simulink model "Copy_of_tests"  (R2024b)
settings: Solver=VariableStepAuto  StartTime=0.0  StopTime=1  RelTol=1e-3  AbsTol=1e-3  EnableMultiTasking=on
values from neighbouring files (symbols this model uses):
  m = obj.Br *obj.volume / obj.mu    [External_Magnet2.m]
  Params = Sim_Param_Setup    [Sim_Open.m]
undefined symbols (not defined in the file or in its folder): X, Y, Z
libraries: sm_lib x171, vrlib x144, nesl_utility x101, matrix_library x91, sharedtransform x12
(part 1 of 9)
settings Model: Creator=user  LastModifiedBy=user
settings SolverCC: AutoScaleAbsTol=off  AlgebraicLoopSolver=TrustRegion  MaxZcPerStep=1
settings DataIOCC: LimitDataPoints=on  MaxDataPoints=10000
settings OptimizationCC: ReuseModelBlockBuffer=off  LifeSpan=inf
settings DebuggingCC: UnconnectedInputMsg=warning  UnconnectedOutputMsg=warning  UnconnectedLineMsg=warning  AllowSymbolicDim=off  SubsystemReferenceDiagnosticForUnitTest=warning  SFUnexpectedBacktrackingDiag=warning  SFNoUnconditionalDefaultTransitionDiag=warning  SFExecutionAtInitializationDiag=none  ArithmeticOperatorsInVariantConditions=warning
settings ModelReferenceCC: EnableRefExpFcnMdlSchedulingChecks=on
settings SFSimCC: SimUseLocalCustomCode=off  CustomCodeUndefinedFunction=UseInterfaceOnly
settings RTWCC: RTWUseLocalCustomCode=off  GPUComputeCapability=3.5  DLArmComputeVersion=19.05
settings CodeAppCC: StateflowObjectComments=on
settings GRTTargetCC: TargetLangStandard=C89/C90 (ANSI)
settings ConfigComp: CovMetricSettings=dw  CovSaveCumulativeToWorkspaceVar=on  CovSaveSingleToWorkspaceVar=on  CovExternalEMLEnable=off  CovSFcnEnable=off
settings SimscapeCC: SimscapeLogType=all  SimscapeLogSimulationStatistics=on  SimscapeLogDataHistory=10000

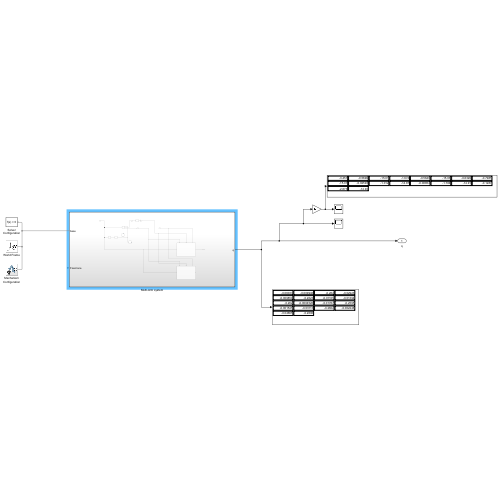
[thumbnail: Simulink's stored preview of the top-level diagram]
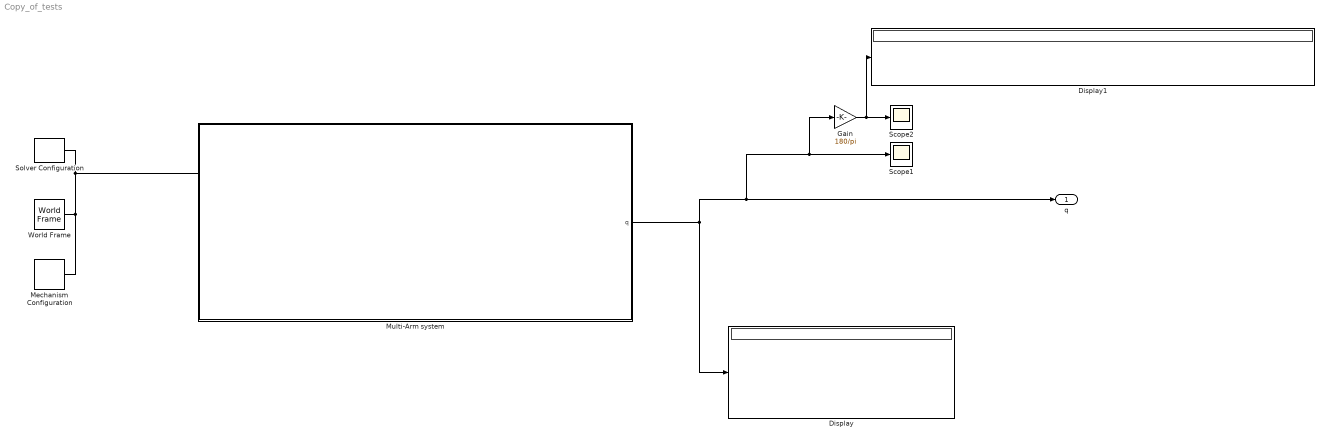
== system Copy_of_tests ==
  Display : Display
  Display1 : Display
  Gain : Gain  Gain=180/pi
  Mechanism Configuration : sm_lib/Utilities/Mechanism Configuration  UniformGravity=Constant  GravityVector=[0 -9.81 0]  GravityVectorUnits=m/s^2  LinearizationDelta=0.001  JointModeTransitionNonlinearIterations=2
  Multi-Arm system : Subsystem
  Scope1 : Scope
  Scope2 : Scope
  Solver Configuration : nesl_utility/Solver Configuration  PhysicalDomain=network_engine_domain  SubClassName=solver  LeftPortType=input  RightPortType=generic  Tones=[]  Harmonics=[]  SimulateNoise=off  Profile=off  UseLocalSampling=off  EnableSwitchedLinearOptims=on  FrequencyDomain=off  UseCCode=off  RelTol=0.001  AbsTol=1e-06  MinStep=1e-09  ToWorkspace=off  RevertToSquareIcSolve=off  NumHomotopyIterations=100  PhasorMode=off  PhasorModeNumHarmonics=1  ConsistencySolver=NEWTON_XTOL_AFTER_FTOL  IndexReductionMethod=DerivativeReplacement  DoDC=off  ResidualTolerance=1e-09  ConsistencyTolSource=GLOBAL  ConsistencyAbsTol=0.001  ConsistencyRelTol=0.001  ConsistencyTolFactor=0.001  UseLocalSolver=off  LocalSolverChoice=NE_BACKWARD_EULER_ADVANCER  ResolveIndetEquations=on  FunctionEvalNumThread=1  LocalSolverSampleTime=0.001  DoFixedCost=off  MaxNonlinIter=3  MaxModeIter=2  ComputeImpulses=off  ImpulseIterations=2  LinearAlgebra=Sparse  LinearAlgebraNumThread=0  EquationFormulation=NE_TIME_EF  DelaysMemoryBudget=1024  AutomaticFiltering=on  FilteringTimeConstant=0.001  PartitionStorageMethod=AS_NEEDED  PartitionMemoryBudget=1024  PartitionMethod=FAST  MultibodyUseLocalSolver=off  MultibodyLocalSolverChoice=ODE1  MultibodyLocalSolverSampleTime=0.001
  World Frame : sm_lib/Frames and Transforms/World Frame
  q : Outport
  wires:
  Gain/1 -> Display1/1, Scope2/1
  Multi-Arm system/1(q) -> Gain/1, Scope1/1, q/1, Display/1
  connections:
  Mechanism Configuration/RConn1 -- Solver Configuration/RConn1 -- Multi-Arm system/LConn1 -- World Frame/RConn1

== system Copy_of_tests/Multi-Arm system ==
  Brick Solid : sm_lib/Body Elements/Brick Solid  BrickDimensions=[5 20 20]  BrickDimensionsUnits=mm  ExportEntireGeometry=off  InertiaType=CalculateFromGeometry  BasedOnType=Density  Density=1000  DensityUnits=kg/m^3  Mass=1  MassUnits=kg  CenterOfMass=[0 0 0]  CenterOfMassUnits=m  MomentsOfInertia=[1 1 1]  MomentsOfInertiaUnits=kg*m^2  ProductsOfInertia=[0 0 0]  ProductsOfInertiaUnits=kg*m^2  GraphicType=FromGeometry  MarkerShape=Sphere  MarkerSize=10  GraphicVisPropType=SimpleVisualProperties  GraphicDiffuseColor=[1 0 0]  GraphicOpacity=1  GraphicSpecularColor=[0.5 0.5 0.5 1.0]  GraphicAmbientColor=[0.15 0.15 0.15 1.0]  GraphicEmissiveColor=[0.0 0.0 0.0 1.0]  GraphicShininess=75  DoExposeReferenceFrame=on  SerializedFrames=<Frames><Frame><Id>Frame1</Id><Value><Name>F1</Name><Origin><Source>GeometricFeature</Source><FeatureName>-x surface</FeatureName></Origin><PrimaryAxis><DefinedDirection>+Z</DefinedDirection><Source>ReferenceFrame</Source><SourceDirection>+Z</SourceDirection><FeatureName></FeatureName></PrimaryAxis><SecondaryAxis><DefinedDirection>+X</DefinedDirection><Source>ReferenceFrame</Source><SourceDirection>+X</SourceDirection><FeatureName></FeatureName></SecondaryAxis></Value></Frame><Frame><Id>Frame2</Id><Value><Name>F2</Name><Origin><Source>GeometricFeature</Source><FeatureName>+x surface</FeatureName></Origin><PrimaryAxis><DefinedDirection>+Z</DefinedDirection><Source>ReferenceFrame</Source><SourceDirection>+Z</SourceDirection><FeatureName></FeatureName></PrimaryAxis><SecondaryAxis><DefinedDirection>+X</DefinedDirection><Source>ReferenceFrame</Source><SourceDirection>+X</SourceDirection><FeatureName></FeatureName></SecondaryAxis></Value></Frame></Frames>
  Brick Solid1 : sm_lib/Body Elements/Brick Solid  BrickDimensions=[5 20 20]  BrickDimensionsUnits=mm  ExportEntireGeometry=off  InertiaType=CalculateFromGeometry  BasedOnType=Density  Density=1000  DensityUnits=kg/m^3  Mass=1  MassUnits=kg  CenterOfMass=[0 0 0]  CenterOfMassUnits=m  MomentsOfInertia=[1 1 1]  MomentsOfInertiaUnits=kg*m^2  ProductsOfInertia=[0 0 0]  ProductsOfInertiaUnits=kg*m^2  GraphicType=FromGeometry  MarkerShape=Sphere  MarkerSize=10  GraphicVisPropType=SimpleVisualProperties  GraphicDiffuseColor=[0 0 1]  GraphicOpacity=1  GraphicSpecularColor=[0.5 0.5 0.5 1.0]  GraphicAmbientColor=[0.15 0.15 0.15 1.0]  GraphicEmissiveColor=[0.0 0.0 0.0 1.0]  GraphicShininess=75  DoExposeReferenceFrame=on  SerializedFrames=<Frames><Frame><Id>Frame1</Id><Value><Name>F1</Name><Origin><Source>GeometricFeature</Source><FeatureName>-x surface</FeatureName></Origin><PrimaryAxis><DefinedDirection>+Z</DefinedDirection><Source>ReferenceFrame</Source><SourceDirection>+Z</SourceDirection><FeatureName></FeatureName></PrimaryAxis><SecondaryAxis><DefinedDirection>+X</DefinedDirection><Source>ReferenceFrame</Source><SourceDirection>+X</SourceDirection><FeatureName></FeatureName></SecondaryAxis></Value></Frame></Frames>
  Gain1 : Gain  Gain=-1*Params.Source_MagnetMagnitude
  PS-Simulink Converter : nesl_utility/PS-Simulink Converter  PhysicalDomain=network_engine_domain  SubClassName=ps_output  LeftPortType=input  RightPortType=output  PseudoPeriodic=off  Frequencies=[]  VectorFormat=inherit  Unit=inherit  AffineConversion=off
  PS-Simulink Converter1 : nesl_utility/PS-Simulink Converter  PhysicalDomain=network_engine_domain  SubClassName=ps_output  LeftPortType=input  RightPortType=output  PseudoPeriodic=off  Frequencies=[]  VectorFormat=inherit  Unit=inherit  AffineConversion=off
  Rigid Transform1 : sm_lib/Frames and Transforms/Rigid Transform  RotationMethod=None  FollAlignAxisA=+X  BaseAlignAxisA=+Y  FollAlignAxisB=+Y  BaseAlignAxisB=+Z  RotationStandardAxis=+Z  RotationAngle=0.0  RotationAngleUnits=deg  RotationArbitraryAxis=[0 0 1]  RotationSequenceAxes=FollowerAxes  RotationSequence=XYX  RotationSequenceAngles=[0 0 0]  RotationSequenceAnglesUnits=deg  RotationMatrix=[1 0 0; 0 1 0; 0 0 1]  Quaternion=[1 0 0 0]  TranslationMethod=Cartesian  TranslationCartesianOffset=[Params.Source_Distance_x Params.Source_Distance_y 0]  TranslationCartesianOffsetUnits=m  TranslationStandardAxis=+X  TranslationStandardOffset=0.1e-3  TranslationStandardOffsetUnits=m  TranslationROffset=0  TranslationROffsetUnits=m  TranslationThetaOffset=0  TranslationThetaOffsetUnits=deg  TranslationZOffset=0  TranslationZOffsetUnits=m
  Rigid Transform2 : sm_lib/Frames and Transforms/Rigid Transform  RotationMethod=StandardAxis  FollAlignAxisA=+X  BaseAlignAxisA=+Y  FollAlignAxisB=+Y  BaseAlignAxisB=+Z  RotationStandardAxis=+Z  RotationAngle=Params.Source_Angle  RotationAngleUnits=deg  RotationArbitraryAxis=[0 0 1]  RotationSequenceAxes=FollowerAxes  RotationSequence=XYX  RotationSequenceAngles=[0 0 0]  RotationSequenceAnglesUnits=deg  RotationMatrix=[1 0 0; 0 1 0; 0 0 1]  Quaternion=[1 0 0 0]  TranslationMethod=None  TranslationCartesianOffset=[Params.Source_Distance_x Params.Source_Distance_y 0]  TranslationCartesianOffsetUnits=m  TranslationStandardAxis=+X  TranslationStandardOffset=0.1e-3  TranslationStandardOffsetUnits=m  TranslationROffset=0  TranslationROffsetUnits=m  TranslationThetaOffset=0  TranslationThetaOffsetUnits=deg  TranslationZOffset=0  TranslationZOffsetUnits=m
  Single_Arm 1 : Subsystem
      settings: PortSchema="{\"entries\":[{\"content\":{\"sides\":[{\"content\":{\"connectorIds\":[\"Out1\"]},\"type\":\"ConnectorPlacement.EquallySpacedRectSide\",\"uuid\":\"aed73cf6-d05b-4742-919d-2a5b7405f7c0\"},{\"content\":{\"connectorIds\":[\"RConn1\"],\"side\":\"RIGHT\"},\"type\":\"ConnectorPlacement.EquallySpacedRectSide\",\"uuid\":\"b6800f08-4bd8-49f5-86ab-f689441aa6b5\"},{\"content\":{\"connectorIds\":[\"LConn1\",\"In1\",\"In2\"],\"side\":\"TOP\"},\"type\":\"ConnectorPlacement.EquallySpacedRectSide\",\"uuid\":\"ec4c69cc-0faf-459d-a169-37761ab2dd6d\"},{\"content\":{\"side\":\"BOTTOM\"},\"type\":\"ConnectorPlacement.EquallySpacedRectSide\",\"uuid\":\"2a21d102-aa49-4e33-81c3-df43061c4ef1\"}]},\"type\":\"ConnectorPlacement.EquallySpacedConnector\",\"uuid\":\"838f12d2-4917-4325-9f22-e0bcefcce707\"}],\"packageUris\":[\"http://schema.mathworks.com/mf0/Connector/R2020b\"],\"version\":\"1.0\"}"
  Single_Arm 2 : Subsystem
      settings: PortSchema="{\"entries\":[{\"content\":{\"sides\":[{\"content\":{\"connectorIds\":[\"Out1\"]},\"type\":\"ConnectorPlacement.EquallySpacedRectSide\",\"uuid\":\"aed73cf6-d05b-4742-919d-2a5b7405f7c0\"},{\"content\":{\"connectorIds\":[\"RConn1\"],\"side\":\"RIGHT\"},\"type\":\"ConnectorPlacement.EquallySpacedRectSide\",\"uuid\":\"b6800f08-4bd8-49f5-86ab-f689441aa6b5\"},{\"content\":{\"connectorIds\":[\"LConn1\",\"In1\",\"In2\"],\"side\":\"TOP\"},\"type\":\"ConnectorPlacement.EquallySpacedRectSide\",\"uuid\":\"ec4c69cc-0faf-459d-a169-37761ab2dd6d\"},{\"content\":{\"side\":\"BOTTOM\"},\"type\":\"ConnectorPlacement.EquallySpacedRectSide\",\"uuid\":\"2a21d102-aa49-4e33-81c3-df43061c4ef1\"}]},\"type\":\"ConnectorPlacement.EquallySpacedConnector\",\"uuid\":\"838f12d2-4917-4325-9f22-e0bcefcce707\"}],\"packageUris\":[\"http://schema.mathworks.com/mf0/Connector/R2020b\"],\"version\":\"1.0\"}"
  Submatrix : matrix_library/Submatrix  RowSpan=Range of rows  RowStartMode=First  RowStartIndex=1  RowEndMode=Last  RowEndIndex=1  ColSpan=One column  ColStartMode=First  ColStartIndex=1  ColEndMode=Last  ColEndIndex=1
  Transform Sensor : sm_lib/Frames and Transforms/Transform Sensor  MeasurementFrame=Base  RotationSequence=XYX  SenseAngle=off  SenseAxis=off  SenseQ=off  SenseR=on  SenseRotationSequence=off  SenseOmegaX=off  SenseOmegaY=off  SenseOmegaZ=off  SenseOmega=off  SenseQDot=off  SenseRDot=off  SenseRotationSequenceDot=off  SenseAlphaX=off  SenseAlphaY=off  SenseAlphaZ=off  SenseAlpha=off  SenseQDDot=off  SenseRDDot=off  SenseX=off  SenseY=off  SenseZ=off  SenseXYZ=on  SenseRad=off  SenseAzim=off  SenseDist=off  SenseInc=off  SenseXDot=off  SenseYDot=off  SenseZDot=off  SenseXYZDot=off  SenseRadDot=off  SenseAzimDot=off  SenseDistDot=off  SenseIncDot=off  SenseXDDot=off  SenseYDDot=off  SenseZDDot=off  SenseXYZDDot=off  SenseRadDDot=off  SenseAzimDDot=off  SenseDistDDot=off  SenseIncDDot=off
  base : PMIOPort  Side=Left
  Fixed one : PMIOPort  Port=2  Side=Left
  q : Outport
  wires:
  PS-Simulink Converter1/1 -> Submatrix/1
  Gain1/1 -> Single_Arm 1/1(Source_Moment), Single_Arm 2/1(Source_Moment)
  Submatrix/1 -> Gain1/1
  Single_Arm 1/1(q) -> q/1
  PS-Simulink Converter/1 -> Single_Arm 1/2(Source_Pos), Single_Arm 2/2(Source_Pos)
  connections:
  Brick Solid/LConn2 -- Transform Sensor/RConn1 -- Brick Solid1/LConn1
  Rigid Transform1/RConn1 -- Rigid Transform2/LConn1
  Rigid Transform2/RConn1 -- Brick Solid/LConn1
  Single_Arm 1/LConn1 -- Fixed one/RConn1 -- Single_Arm 2/LConn1
  base/RConn1 -- Single_Arm 2/RConn1 -- Single_Arm 1/RConn1 -- Rigid Transform1/LConn1 -- Transform Sensor/LConn1
  Transform Sensor/RConn3 -- PS-Simulink Converter/LConn1
  PS-Simulink Converter1/LConn1 -- Transform Sensor/RConn2

== system Copy_of_tests/Multi-Arm system/Single_Arm 1 ==
  Source_Moment : Inport
  Source_Pos : Inport  Port=2
  Mux : Mux  Inputs=6
  PS-Simulink Converter{,1..5} (6 alike) : nesl_utility/PS-Simulink Converter  PhysicalDomain=network_engine_domain  SubClassName=ps_output  LeftPortType=input  RightPortType=output  PseudoPeriodic=off  Frequencies=[]  VectorFormat=inherit  Unit=inherit  AffineConversion=off
  Plate_0 : Subsystem
  Plate_1 : Subsystem
      settings: PortSchema="{\"entries\":[{\"content\":{\"sides\":[{\"content\":{\"connectorIds\":[\"LConn1\"]},\"type\":\"ConnectorPlacement.EquallySpacedRectSide\",\"uuid\":\"d3209e73-b1b0-400d-bb69-5c2c223e1cf5\"},{\"content\":{\"connectorIds\":[\"RConn1\"],\"side\":\"RIGHT\"},\"type\":\"ConnectorPlacement.EquallySpacedRectSide\",\"uuid\":\"f1a30951-4015-44b6-8cd5-c465137d5200\"},{\"content\":{\"connectorIds\":[\"In1\",\"In2\",\"In3\",\"In4\",\"In5\",\"In6\",\"In7\",\"In8\",\"In9\",\"In10\",\"Out1\",\"Out2\"],\"side\":\"TOP\"},\"type\":\"ConnectorPlacement.EquallySpacedRectSide\",\"uuid\":\"858e4eb2-ea22-4c31-a0a7-90acc6749235\"},{\"content\":{\"connectorIds\":[\"In11\",\"In12\"],\"side\":\"BOTTOM\"},\"type\":\"ConnectorPlacement.EquallySpacedRectSide\",\"uuid\":\"4614ed4f-637f-4a9b-aac4-e5064df79866\"}]},\"type\":\"ConnectorPlacement.EquallySpacedConnector\",\"uuid\":\"0376ba42-8dd9-4ddf-9e80-cb6449970d36\"}],\"packageUris\":[\"http://schema.mathworks.com/mf0/Connector/R2020b\"],\"version\":\"1.0\"}"
  Plate_2 : Subsystem
      settings: PortSchema="{\"entries\":[{\"content\":{\"sides\":[{\"content\":{\"connectorIds\":[\"LConn1\"]},\"type\":\"ConnectorPlacement.EquallySpacedRectSide\",\"uuid\":\"ec18759c-59e4-4a78-8a02-c5f79d16e625\"},{\"content\":{\"connectorIds\":[\"RConn1\"],\"side\":\"RIGHT\"},\"type\":\"ConnectorPlacement.EquallySpacedRectSide\",\"uuid\":\"7dbb223b-0b69-4dcf-bc3d-f54c7924a0b4\"},{\"content\":{\"connectorIds\":[\"In1\",\"In2\",\"In3\",\"In4\",\"In5\",\"In6\",\"In7\",\"In8\",\"Out1\",\"Out2\",\"In9\",\"In10\"],\"side\":\"TOP\"},\"type\":\"ConnectorPlacement.EquallySpacedRectSide\",\"uuid\":\"897f1654-1cd8-4ed9-9f75-2958da94a55c\"},{\"content\":{\"connectorIds\":[\"In11\",\"In12\"],\"side\":\"BOTTOM\"},\"type\":\"ConnectorPlacement.EquallySpacedRectSide\",\"uuid\":\"7ed320ae-75a8-4e52-84a2-f6626d5c5d01\"}]},\"type\":\"ConnectorPlacement.EquallySpacedConnector\",\"uuid\":\"b5c764c2-43a6-4160-9b0c-e997344b52fc\"}],\"packageUris\":[\"http://schema.mathworks.com/mf0/Connector/R2020b\"],\"version\":\"1.0\"}"
  Plate_3 : Subsystem
      settings: PortSchema="{\"entries\":[{\"content\":{\"sides\":[{\"content\":{\"connectorIds\":[\"LConn1\"]},\"type\":\"ConnectorPlacement.EquallySpacedRectSide\",\"uuid\":\"659d4c74-debd-4236-880d-faa78149b6ae\"},{\"content\":{\"connectorIds\":[\"RConn1\"],\"side\":\"RIGHT\"},\"type\":\"ConnectorPlacement.EquallySpacedRectSide\",\"uuid\":\"7acc4d0a-33e4-40af-a3d8-89f29cefab0d\"},{\"content\":{\"connectorIds\":[\"In1\",\"In2\",\"In3\",\"In4\",\"In5\",\"In6\",\"Out1\",\"Out2\",\"In7\",\"In8\",\"In9\",\"In10\"],\"side\":\"TOP\"},\"type\":\"ConnectorPlacement.EquallySpacedRectSide\",\"uuid\":\"3f8fe647-c128-4da8-9892-2ef747b61f38\"},{\"content\":{\"connectorIds\":[\"In11\",\"In12\"],\"side\":\"BOTTOM\"},\"type\":\"ConnectorPlacement.EquallySpacedRectSide\",\"uuid\":\"9ec47aaa-5f22-4f0a-90c6-c481dcf8db46\"}]},\"type\":\"ConnectorPlacement.EquallySpacedConnector\",\"uuid\":\"1b26417e-b7bd-4e51-87e9-74b02b81f54b\"}],\"packageUris\":[\"http://schema.mathworks.com/mf0/Connector/R2020b\"],\"version\":\"1.0\"}"
  Plate_4 : Subsystem
      settings: PortSchema="{\"entries\":[{\"content\":{\"sides\":[{\"content\":{\"connectorIds\":[\"LConn1\"]},\"type\":\"ConnectorPlacement.EquallySpacedRectSide\",\"uuid\":\"ec18759c-59e4-4a78-8a02-c5f79d16e625\"},{\"content\":{\"connectorIds\":[\"RConn1\"],\"side\":\"RIGHT\"},\"type\":\"ConnectorPlacement.EquallySpacedRectSide\",\"uuid\":\"7dbb223b-0b69-4dcf-bc3d-f54c7924a0b4\"},{\"content\":{\"connectorIds\":[\"In1\",\"In2\",\"In3\",\"In4\",\"Out1\",\"Out2\",\"In5\",\"In6\",\"In7\",\"In8\",\"In9\",\"In10\"],\"side\":\"TOP\"},\"type\":\"ConnectorPlacement.EquallySpacedRectSide\",\"uuid\":\"897f1654-1cd8-4ed9-9f75-2958da94a55c\"},{\"content\":{\"connectorIds\":[\"In11\",\"In12\"],\"side\":\"BOTTOM\"},\"type\":\"ConnectorPlacement.EquallySpacedRectSide\",\"uuid\":\"3c262aa2-4d18-4ec5-8376-adcb010a8e7d\"}]},\"type\":\"ConnectorPlacement.EquallySpacedConnector\",\"uuid\":\"b5c764c2-43a6-4160-9b0c-e997344b52fc\"}],\"packageUris\":[\"http://schema.mathworks.com/mf0/Connector/R2020b\"],\"version\":\"1.0\"}"
  Plate_5 : Subsystem
      settings: PortSchema="{\"entries\":[{\"content\":{\"sides\":[{\"content\":{\"connectorIds\":[\"LConn1\"]},\"type\":\"ConnectorPlacement.EquallySpacedRectSide\",\"uuid\":\"ec18759c-59e4-4a78-8a02-c5f79d16e625\"},{\"content\":{\"connectorIds\":[\"RConn1\"],\"side\":\"RIGHT\"},\"type\":\"ConnectorPlacement.EquallySpacedRectSide\",\"uuid\":\"7dbb223b-0b69-4dcf-bc3d-f54c7924a0b4\"},{\"content\":{\"connectorIds\":[\"In1\",\"In2\",\"Out1\",\"Out2\",\"In3\",\"In4\",\"In5\",\"In6\",\"In7\",\"In8\",\"In9\",\"In10\"],\"side\":\"TOP\"},\"type\":\"ConnectorPlacement.EquallySpacedRectSide\",\"uuid\":\"897f1654-1cd8-4ed9-9f75-2958da94a55c\"},{\"content\":{\"connectorIds\":[\"In11\",\"In12\"],\"side\":\"BOTTOM\"},\"type\":\"ConnectorPlacement.EquallySpacedRectSide\",\"uuid\":\"5987a4f9-0df9-407c-b6e6-a076c5272fc6\"}]},\"type\":\"ConnectorPlacement.EquallySpacedConnector\",\"uuid\":\"b5c764c2-43a6-4160-9b0c-e997344b52fc\"}],\"packageUris\":[\"http://schema.mathworks.com/mf0/Connector/R2020b\"],\"version\":\"1.0\"}"
  Plate_6 : Subsystem
      settings: PortSchema="{\"entries\":[{\"content\":{\"sides\":[{\"content\":{\"connectorIds\":[\"LConn1\"]},\"type\":\"ConnectorPlacement.EquallySpacedRectSide\",\"uuid\":\"ec18759c-59e4-4a78-8a02-c5f79d16e625\"},{\"content\":{\"connectorIds\":[\"RConn1\"],\"side\":\"RIGHT\"},\"type\":\"ConnectorPlacement.EquallySpacedRectSide\",\"uuid\":\"7dbb223b-0b69-4dcf-bc3d-f54c7924a0b4\"},{\"content\":{\"connectorIds\":[\"Out1\",\"Out2\",\"In1\",\"In2\",\"In3\",\"In4\",\"In5\",\"In6\",\"In7\",\"In8\",\"In9\",\"In10\"],\"side\":\"TOP\"},\"type\":\"ConnectorPlacement.EquallySpacedRectSide\",\"uuid\":\"897f1654-1cd8-4ed9-9f75-2958da94a55c\"},{\"content\":{\"connectorIds\":[\"In11\",\"In12\"],\"side\":\"BOTTOM\"},\"type\":\"ConnectorPlacement.EquallySpacedRectSide\",\"uuid\":\"c3ba0d0a-cbda-4d2d-b1e9-4fbf79d48483\"}]},\"type\":\"ConnectorPlacement.EquallySpacedConnector\",\"uuid\":\"b5c764c2-43a6-4160-9b0c-e997344b52fc\"}],\"packageUris\":[\"http://schema.mathworks.com/mf0/Connector/R2020b\"],\"version\":\"1.0\"}"
  Quaternions to Rotation Angles{,1..5} (6 alike) : sharedtransform/Quaternions to Rotation Angles  rotationOrder=ZYX  aMode=aMode
  Rigid Transform{1..12} (12 alike) : sm_lib/Frames and Transforms/Rigid Transform  RotationMethod=None  FollAlignAxisA=+X  BaseAlignAxisA=+Y  FollAlignAxisB=+Y  BaseAlignAxisB=+Z  RotationStandardAxis=+Z  RotationAngle=0.0  RotationAngleUnits=deg  RotationArbitraryAxis=[0 0 1]  RotationSequenceAxes=FollowerAxes  RotationSequence=XYX  RotationSequenceAngles=[0 0 0]  RotationSequenceAnglesUnits=deg  RotationMatrix=[1 0 0; 0 1 0; 0 0 1]  Quaternion=[1 0 0 0]  TranslationMethod=StandardAxis  TranslationCartesianOffset=[0 0 0]  TranslationCartesianOffsetUnits=m  TranslationStandardAxis=+X  TranslationStandardOffset=0.1e-3  TranslationStandardOffsetUnits=m  TranslationROffset=0  TranslationROffsetUnits=m  TranslationThetaOffset=0  TranslationThetaOffsetUnits=deg  TranslationZOffset=0  TranslationZOffsetUnits=m
  Spherical Joint{,1..5} (6 alike) : sm_lib/Joints/Spherical Joint  JointMode=Normal  CompositeWrenchDir=FollowerOnBase  CompositeWrenchFrame=BaseFrame  SenseConstraintForce=off  SenseConstraintTorque=off  SenseTotalForce=off  SenseTotalTorque=off  PositionTargetSpecify=off  PositionTargetPriority=High  PositionTargetRotationMethod=None  PositionTargetFollAlignAxisA=+X  PositionTargetBaseAlignAxisA=+Y  PositionTargetFollAlignAxisB=+Y  PositionTargetBaseAlignAxisB=+Z  PositionTargetRotationStandardAxis=+Z  PositionTargetRotationAngle=0  PositionTargetRotationAngleUnits=deg  PositionTargetRotationArbitraryAxis=[0 0 1]  PositionTargetRotationSequenceAxes=FollowerAxes  PositionTargetRotationSequence=XYX  PositionTargetRotationSequenceAngles=[0 0 0]  PositionTargetRotationSequenceAnglesUnits=deg  PositionTargetRotationMatrix=[1 0 0;0 1 0;0 0 1]  PositionTargetQuaternion=[1 0 0 0]  VelocityTargetSpecify=off  VelocityTargetPriority=High  VelocityTargetValue=[0 0 0]  VelocityTargetValueUnits=deg/s  VelocityTargetInFollowerFrame=on  EqPosRotationMethod=None  EqPosFollAlignAxisA=+X  EqPosBaseAlignAxisA=+Y  EqPosFollAlignAxisB=+Y  EqPosBaseAlignAxisB=+Z  EqPosRotationStandardAxis=+Z  EqPosRotationAngle=0  EqPosRotationAngleUnits=deg  EqPosRotationArbitraryAxis=[0 0 1]  EqPosRotationSequenceAxes=FollowerAxes  EqPosRotationSequence=XYX  EqPosRotationSequenceAngles=[0 0 0]  EqPosRotationSequenceAnglesUnits=deg  EqPosRotationMatrix=[1 0 0;0 1 0;0 0 1]  EqPosQuaternion=[1 0 0 0]  SpringStiffness=Params.Stiffness  SpringStiffnessUnits=N*m/deg  DampingCoefficient=Params.Damping  DampingCoefficientUnits=N*m/(deg/s)  LowerLimitSpecify=off  LowerLimitBound=15  LowerLimitBoundUnits=deg  LowerLimitStiffness=1e4  LowerLimitStiffnessUnits=N*m/deg  LowerLimitDamping=10  LowerLimitDampingUnits=N*m/(deg/s)  LowerLimitTransitionRegionWidth=0.1  LowerLimitTransitionRegionWidthUnits=deg  UpperLimitSpecify=off  UpperLimitBound=45  UpperLimitBoundUnits=deg  UpperLimitStiffness=1e4  UpperLimitStiffnessUnits=N*m/deg  UpperLimitDamping=10  UpperLimitDampingUnits=N*m/(deg/s)  UpperLimitTransitionRegionWidth=0.1  UpperLimitTransitionRegionWidthUnits=deg  TorqueActuationMode=NoTorque  ActuateTorqueX=off  ActuateTorqueY=off  ActuateTorqueZ=off  ActuateTorque=off  ActuationFrame=BaseFrame  SensePosition=on  SenseVelocityX=off  SenseVelocityY=off  SenseVelocityZ=off  SenseVelocity=off  SenseAccelerationX=off  SenseAccelerationY=off  SenseAccelerationZ=off  SenseAcceleration=off  SenseLowerLimitTorqueMag=off  SenseUpperLimitTorqueMag=off  SensingFrame=BaseFrame
  Fixed one : PMIOPort  Side=Left
  base : PMIOPort  Port=2  Side=Right
  q : Outport
  wires:
  PS-Simulink Converter/1 -> Quaternions to Rotation Angles/1
  PS-Simulink Converter1/1 -> Quaternions to Rotation Angles1/1
  PS-Simulink Converter2/1 -> Quaternions to Rotation Angles2/1
  PS-Simulink Converter3/1 -> Quaternions to Rotation Angles3/1
  PS-Simulink Converter5/1 -> Quaternions to Rotation Angles5/1
  PS-Simulink Converter4/1 -> Quaternions to Rotation Angles4/1
  Mux/1 -> q/1
  Plate_2/1(Pos_Plate2) -> Plate_6/7(Pos_Plate2), Plate_5/7(Pos_Plate2), Plate_4/7(Pos_Plate2), Plate_3/7(Pos_Plate2), Plate_1/9(Pos_Plate2)
  Plate_2/2(M2) -> Plate_6/8(M2), Plate_5/8(M2), Plate_4/8(M2), Plate_3/8(M2), Plate_1/10(M2)
  Plate_1/2(M1) -> Plate_6/10(M1), Plate_5/10(M1), Plate_4/10(M1), Plate_3/10(M1), Plate_2/10(M1)
  Plate_1/1(Pos_Plate1) -> Plate_6/9(Pos_Plate1), Plate_5/9(Pos_Plate1), Plate_4/9(Pos_Plate1), Plate_3/9(Pos_Plate1), Plate_2/9(Pos_Plate1)
  Plate_3/2(M3) -> Plate_6/6(M3), Plate_5/6(M3), Plate_4/6(M3), Plate_2/8(M3), Plate_1/8(M3)
  Plate_3/1(Pos_Plate3) -> Plate_6/5(Pos_Plate3), Plate_5/5(Pos_Plate3), Plate_4/5(Pos_Plate3), Plate_2/7(Pos_Plate3), Plate_1/7(Pos_Plate3)
  Plate_4/2(M4) -> Plate_6/4(M4), Plate_5/4(M4), Plate_3/6(M4), Plate_2/6(M4), Plate_1/6(M4)
  Plate_4/1(Pos_Plate4) -> Plate_6/3(Pos_Plate4), Plate_5/3(Pos_Plate4), Plate_3/5(Pos_Plate4), Plate_2/5(Pos_Plate4), Plate_1/5(Pos_Plate4)
  Plate_5/2(M5) -> Plate_6/2(M5), Plate_4/4(M5), Plate_3/4(M5), Plate_2/4(M5), Plate_1/4(M5)
  Plate_5/1(Pos_Plate5) -> Plate_6/1(Pos_Plate5), Plate_4/3(Pos_Plate5), Plate_3/3(Pos_Plate5), Plate_2/3(Pos_Plate5), Plate_1/3(Pos_Plate5)
  Plate_6/2(M6) -> Plate_5/2(M6), Plate_4/2(M6), Plate_3/2(M6), Plate_2/2(M6), Plate_1/2(M6)
  Plate_6/1(Pos_Plate6) -> Plate_5/1(Pos_Plate6), Plate_4/1(Pos_Plate6), Plate_3/1(Pos_Plate6), Plate_2/1(Pos_Plate6), Plate_1/1(Pos_Plate6)
  Quaternions to Rotation Angles/1 -> Mux/1
  Quaternions to Rotation Angles1/1 -> Mux/2
  Quaternions to Rotation Angles2/1 -> Mux/3
  Quaternions to Rotation Angles3/1 -> Mux/4
  Quaternions to Rotation Angles4/1 -> Mux/5
  Quaternions to Rotation Angles5/1 -> Mux/6
  Source_Moment/1 -> Plate_6/12(Source_Moment), Plate_5/12(Source_Moment), Plate_4/12(Source_Moment), Plate_3/12(Source_Moment), Plate_2/12(Source_Moment), Plate_1/12(Source_Moment)
  Source_Pos/1 -> Plate_6/11(Source_Pos), Plate_5/11(Source_Pos), Plate_4/11(Source_Pos), Plate_3/11(Source_Pos), Plate_2/11(Source_Pos), Plate_1/11(Source_Pos)
  connections:
  Rigid Transform11/RConn1 -- Plate_6/RConn1
  Spherical Joint1/LConn1 -- Rigid Transform3/RConn1
  Spherical Joint5/LConn1 -- Rigid Transform12/RConn1
  Rigid Transform2/LConn1 -- Spherical Joint/RConn1
  Rigid Transform11/LConn1 -- Spherical Joint5/RConn1
  Rigid Transform10/RConn1 -- Plate_5/RConn1
  Rigid Transform10/LConn1 -- Spherical Joint4/RConn1
  Rigid Transform4/LConn1 -- Spherical Joint1/RConn1
  Rigid Transform8/RConn1 -- Plate_4/RConn1
  Spherical Joint4/LConn1 -- Rigid Transform9/RConn1
  Plate_4/LConn1 -- Rigid Transform9/LConn1
  Spherical Joint3/LConn1 -- Rigid Transform7/RConn1
  Rigid Transform6/RConn1 -- Plate_3/RConn1
  Rigid Transform8/LConn1 -- Spherical Joint3/RConn1
  Plate_3/LConn1 -- Rigid Transform7/LConn1
  Plate_0/LConn1 -- Rigid Transform1/LConn1
  Spherical Joint/LConn1 -- Rigid Transform1/RConn1
  Plate_2/LConn1 -- Rigid Transform5/LConn1
  Plate_1/LConn1 -- Rigid Transform3/LConn1
  Plate_5/LConn1 -- Rigid Transform12/LConn1
  Rigid Transform4/RConn1 -- Plate_2/RConn1
  Spherical Joint2/LConn1 -- Rigid Transform5/RConn1
  Rigid Transform6/LConn1 -- Spherical Joint2/RConn1
  Rigid Transform2/RConn1 -- Plate_1/RConn1
  Plate_6/LConn1 -- Fixed one/RConn1
  base/RConn1 -- Plate_0/RConn1
  Spherical Joint/RConn2 -- PS-Simulink Converter/LConn1
  Spherical Joint1/RConn2 -- PS-Simulink Converter1/LConn1
  Spherical Joint2/RConn2 -- PS-Simulink Converter2/LConn1
  Spherical Joint3/RConn2 -- PS-Simulink Converter3/LConn1
  Spherical Joint4/RConn2 -- PS-Simulink Converter4/LConn1
  Spherical Joint5/RConn2 -- PS-Simulink Converter5/LConn1

== system Copy_of_tests/Multi-Arm system/Single_Arm 2 ==
  Source_Moment : Inport
  Source_Pos : Inport  Port=2
  Mux : Mux  Inputs=6
  PS-Simulink Converter{,1..5} (6 alike) : nesl_utility/PS-Simulink Converter  PhysicalDomain=network_engine_domain  SubClassName=ps_output  LeftPortType=input  RightPortType=output  PseudoPeriodic=off  Frequencies=[]  VectorFormat=inherit  Unit=inherit  AffineConversion=off
  Plate_0 : Subsystem
  Plate_1 : Subsystem
      settings: PortSchema="{\"entries\":[{\"content\":{\"sides\":[{\"content\":{\"connectorIds\":[\"LConn1\"]},\"type\":\"ConnectorPlacement.EquallySpacedRectSide\",\"uuid\":\"d3209e73-b1b0-400d-bb69-5c2c223e1cf5\"},{\"content\":{\"connectorIds\":[\"RConn1\"],\"side\":\"RIGHT\"},\"type\":\"ConnectorPlacement.EquallySpacedRectSide\",\"uuid\":\"f1a30951-4015-44b6-8cd5-c465137d5200\"},{\"content\":{\"connectorIds\":[\"In1\",\"In2\",\"In3\",\"In4\",\"In5\",\"In6\",\"In7\",\"In8\",\"In9\",\"In10\",\"Out1\",\"Out2\"],\"side\":\"TOP\"},\"type\":\"ConnectorPlacement.EquallySpacedRectSide\",\"uuid\":\"858e4eb2-ea22-4c31-a0a7-90acc6749235\"},{\"content\":{\"connectorIds\":[\"In11\",\"In12\"],\"side\":\"BOTTOM\"},\"type\":\"ConnectorPlacement.EquallySpacedRectSide\",\"uuid\":\"4614ed4f-637f-4a9b-aac4-e5064df79866\"}]},\"type\":\"ConnectorPlacement.EquallySpacedConnector\",\"uuid\":\"0376ba42-8dd9-4ddf-9e80-cb6449970d36\"}],\"packageUris\":[\"http://schema.mathworks.com/mf0/Connector/R2020b\"],\"version\":\"1.0\"}"
  Plate_2 : Subsystem
      settings: PortSchema="{\"entries\":[{\"content\":{\"sides\":[{\"content\":{\"connectorIds\":[\"LConn1\"]},\"type\":\"ConnectorPlacement.EquallySpacedRectSide\",\"uuid\":\"ec18759c-59e4-4a78-8a02-c5f79d16e625\"},{\"content\":{\"connectorIds\":[\"RConn1\"],\"side\":\"RIGHT\"},\"type\":\"ConnectorPlacement.EquallySpacedRectSide\",\"uuid\":\"7dbb223b-0b69-4dcf-bc3d-f54c7924a0b4\"},{\"content\":{\"connectorIds\":[\"In1\",\"In2\",\"In3\",\"In4\",\"In5\",\"In6\",\"In7\",\"In8\",\"Out1\",\"Out2\",\"In9\",\"In10\"],\"side\":\"TOP\"},\"type\":\"ConnectorPlacement.EquallySpacedRectSide\",\"uuid\":\"897f1654-1cd8-4ed9-9f75-2958da94a55c\"},{\"content\":{\"connectorIds\":[\"In11\",\"In12\"],\"side\":\"BOTTOM\"},\"type\":\"ConnectorPlacement.EquallySpacedRectSide\",\"uuid\":\"7ed320ae-75a8-4e52-84a2-f6626d5c5d01\"}]},\"type\":\"ConnectorPlacement.EquallySpacedConnector\",\"uuid\":\"b5c764c2-43a6-4160-9b0c-e997344b52fc\"}],\"packageUris\":[\"http://schema.mathworks.com/mf0/Connector/R2020b\"],\"version\":\"1.0\"}"
  Plate_3 : Subsystem
      settings: PortSchema="{\"entries\":[{\"content\":{\"sides\":[{\"content\":{\"connectorIds\":[\"LConn1\"]},\"type\":\"ConnectorPlacement.EquallySpacedRectSide\",\"uuid\":\"659d4c74-debd-4236-880d-faa78149b6ae\"},{\"content\":{\"connectorIds\":[\"RConn1\"],\"side\":\"RIGHT\"},\"type\":\"ConnectorPlacement.EquallySpacedRectSide\",\"uuid\":\"7acc4d0a-33e4-40af-a3d8-89f29cefab0d\"},{\"content\":{\"connectorIds\":[\"In1\",\"In2\",\"In3\",\"In4\",\"In5\",\"In6\",\"Out1\",\"Out2\",\"In7\",\"In8\",\"In9\",\"In10\"],\"side\":\"TOP\"},\"type\":\"ConnectorPlacement.EquallySpacedRectSide\",\"uuid\":\"3f8fe647-c128-4da8-9892-2ef747b61f38\"},{\"content\":{\"connectorIds\":[\"In11\",\"In12\"],\"side\":\"BOTTOM\"},\"type\":\"ConnectorPlacement.EquallySpacedRectSide\",\"uuid\":\"9ec47aaa-5f22-4f0a-90c6-c481dcf8db46\"}]},\"type\":\"ConnectorPlacement.EquallySpacedConnector\",\"uuid\":\"1b26417e-b7bd-4e51-87e9-74b02b81f54b\"}],\"packageUris\":[\"http://schema.mathworks.com/mf0/Connector/R2020b\"],\"version\":\"1.0\"}"
  Plate_4 : Subsystem
      settings: PortSchema="{\"entries\":[{\"content\":{\"sides\":[{\"content\":{\"connectorIds\":[\"LConn1\"]},\"type\":\"ConnectorPlacement.EquallySpacedRectSide\",\"uuid\":\"ec18759c-59e4-4a78-8a02-c5f79d16e625\"},{\"content\":{\"connectorIds\":[\"RConn1\"],\"side\":\"RIGHT\"},\"type\":\"ConnectorPlacement.EquallySpacedRectSide\",\"uuid\":\"7dbb223b-0b69-4dcf-bc3d-f54c7924a0b4\"},{\"content\":{\"connectorIds\":[\"In1\",\"In2\",\"In3\",\"In4\",\"Out1\",\"Out2\",\"In5\",\"In6\",\"In7\",\"In8\",\"In9\",\"In10\"],\"side\":\"TOP\"},\"type\":\"ConnectorPlacement.EquallySpacedRectSide\",\"uuid\":\"897f1654-1cd8-4ed9-9f75-2958da94a55c\"},{\"content\":{\"connectorIds\":[\"In11\",\"In12\"],\"side\":\"BOTTOM\"},\"type\":\"ConnectorPlacement.EquallySpacedRectSide\",\"uuid\":\"3c262aa2-4d18-4ec5-8376-adcb010a8e7d\"}]},\"type\":\"ConnectorPlacement.EquallySpacedConnector\",\"uuid\":\"b5c764c2-43a6-4160-9b0c-e997344b52fc\"}],\"packageUris\":[\"http://schema.mathworks.com/mf0/Connector/R2020b\"],\"version\":\"1.0\"}"
  Plate_5 : Subsystem
      settings: PortSchema="{\"entries\":[{\"content\":{\"sides\":[{\"content\":{\"connectorIds\":[\"LConn1\"]},\"type\":\"ConnectorPlacement.EquallySpacedRectSide\",\"uuid\":\"ec18759c-59e4-4a78-8a02-c5f79d16e625\"},{\"content\":{\"connectorIds\":[\"RConn1\"],\"side\":\"RIGHT\"},\"type\":\"ConnectorPlacement.EquallySpacedRectSide\",\"uuid\":\"7dbb223b-0b69-4dcf-bc3d-f54c7924a0b4\"},{\"content\":{\"connectorIds\":[\"In1\",\"In2\",\"Out1\",\"Out2\",\"In3\",\"In4\",\"In5\",\"In6\",\"In7\",\"In8\",\"In9\",\"In10\"],\"side\":\"TOP\"},\"type\":\"ConnectorPlacement.EquallySpacedRectSide\",\"uuid\":\"897f1654-1cd8-4ed9-9f75-2958da94a55c\"},{\"content\":{\"connectorIds\":[\"In11\",\"In12\"],\"side\":\"BOTTOM\"},\"type\":\"ConnectorPlacement.EquallySpacedRectSide\",\"uuid\":\"5987a4f9-0df9-407c-b6e6-a076c5272fc6\"}]},\"type\":\"ConnectorPlacement.EquallySpacedConnector\",\"uuid\":\"b5c764c2-43a6-4160-9b0c-e997344b52fc\"}],\"packageUris\":[\"http://schema.mathworks.com/mf0/Connector/R2020b\"],\"version\":\"1.0\"}"
  Plate_6 : Subsystem
      settings: PortSchema="{\"entries\":[{\"content\":{\"sides\":[{\"content\":{\"connectorIds\":[\"LConn1\"]},\"type\":\"ConnectorPlacement.EquallySpacedRectSide\",\"uuid\":\"ec18759c-59e4-4a78-8a02-c5f79d16e625\"},{\"content\":{\"connectorIds\":[\"RConn1\"],\"side\":\"RIGHT\"},\"type\":\"ConnectorPlacement.EquallySpacedRectSide\",\"uuid\":\"7dbb223b-0b69-4dcf-bc3d-f54c7924a0b4\"},{\"content\":{\"connectorIds\":[\"Out1\",\"Out2\",\"In1\",\"In2\",\"In3\",\"In4\",\"In5\",\"In6\",\"In7\",\"In8\",\"In9\",\"In10\"],\"side\":\"TOP\"},\"type\":\"ConnectorPlacement.EquallySpacedRectSide\",\"uuid\":\"897f1654-1cd8-4ed9-9f75-2958da94a55c\"},{\"content\":{\"connectorIds\":[\"In11\",\"In12\"],\"side\":\"BOTTOM\"},\"type\":\"ConnectorPlacement.EquallySpacedRectSide\",\"uuid\":\"c3ba0d0a-cbda-4d2d-b1e9-4fbf79d48483\"}]},\"type\":\"ConnectorPlacement.EquallySpacedConnector\",\"uuid\":\"b5c764c2-43a6-4160-9b0c-e997344b52fc\"}],\"packageUris\":[\"http://schema.mathworks.com/mf0/Connector/R2020b\"],\"version\":\"1.0\"}"
  Quaternions to Rotation Angles{,1..5} (6 alike) : sharedtransform/Quaternions to Rotation Angles  rotationOrder=ZYX  aMode=aMode
  Rigid Transform{1..12} (12 alike) : sm_lib/Frames and Transforms/Rigid Transform  RotationMethod=None  FollAlignAxisA=+X  BaseAlignAxisA=+Y  FollAlignAxisB=+Y  BaseAlignAxisB=+Z  RotationStandardAxis=+Z  RotationAngle=0.0  RotationAngleUnits=deg  RotationArbitraryAxis=[0 0 1]  RotationSequenceAxes=FollowerAxes  RotationSequence=XYX  RotationSequenceAngles=[0 0 0]  RotationSequenceAnglesUnits=deg  RotationMatrix=[1 0 0; 0 1 0; 0 0 1]  Quaternion=[1 0 0 0]  TranslationMethod=StandardAxis  TranslationCartesianOffset=[0 0 0]  TranslationCartesianOffsetUnits=m  TranslationStandardAxis=+X  TranslationStandardOffset=0.1e-3  TranslationStandardOffsetUnits=m  TranslationROffset=0  TranslationROffsetUnits=m  TranslationThetaOffset=0  TranslationThetaOffsetUnits=deg  TranslationZOffset=0  TranslationZOffsetUnits=m
  Rigid Transform13 : sm_lib/Frames and Transforms/Rigid Transform  RotationMethod=None  FollAlignAxisA=+X  BaseAlignAxisA=+Y  FollAlignAxisB=+Y  BaseAlignAxisB=+Z  RotationStandardAxis=+Z  RotationAngle=0.0  RotationAngleUnits=deg  RotationArbitraryAxis=[0 0 1]  RotationSequenceAxes=FollowerAxes  RotationSequence=XYX  RotationSequenceAngles=[0 0 0]  RotationSequenceAnglesUnits=deg  RotationMatrix=[1 0 0; 0 1 0; 0 0 1]  Quaternion=[1 0 0 0]  TranslationMethod=StandardAxis  TranslationCartesianOffset=[0 0 0]  TranslationCartesianOffsetUnits=m  TranslationStandardAxis=+Y  TranslationStandardOffset=-1.5e-3  TranslationStandardOffsetUnits=m  TranslationROffset=0  TranslationROffsetUnits=m  TranslationThetaOffset=0  TranslationThetaOffsetUnits=deg  TranslationZOffset=0  TranslationZOffsetUnits=m
  Rigid Transform14 : sm_lib/Frames and Transforms/Rigid Transform  RotationMethod=StandardAxis  FollAlignAxisA=+X  BaseAlignAxisA=+Y  FollAlignAxisB=+Y  BaseAlignAxisB=+Z  RotationStandardAxis=+X  RotationAngle=180  RotationAngleUnits=deg  RotationArbitraryAxis=[0 0 1]  RotationSequenceAxes=FollowerAxes  RotationSequence=XYX  RotationSequenceAngles=[0 0 0]  RotationSequenceAnglesUnits=deg  RotationMatrix=[1 0 0; 0 1 0; 0 0 1]  Quaternion=[1 0 0 0]  TranslationMethod=None  TranslationCartesianOffset=[0 0 0]  TranslationCartesianOffsetUnits=m  TranslationStandardAxis=+Y  TranslationStandardOffset=-1.5e-3  TranslationStandardOffsetUnits=m  TranslationROffset=0  TranslationROffsetUnits=m  TranslationThetaOffset=0  TranslationThetaOffsetUnits=deg  TranslationZOffset=0  TranslationZOffsetUnits=m
  Spherical Joint{,1..5} (6 alike) : sm_lib/Joints/Spherical Joint  JointMode=Normal  CompositeWrenchDir=FollowerOnBase  CompositeWrenchFrame=BaseFrame  SenseConstraintForce=off  SenseConstraintTorque=off  SenseTotalForce=off  SenseTotalTorque=off  PositionTargetSpecify=off  PositionTargetPriority=High  PositionTargetRotationMethod=None  PositionTargetFollAlignAxisA=+X  PositionTargetBaseAlignAxisA=+Y  PositionTargetFollAlignAxisB=+Y  PositionTargetBaseAlignAxisB=+Z  PositionTargetRotationStandardAxis=+Z  PositionTargetRotationAngle=0  PositionTargetRotationAngleUnits=deg  PositionTargetRotationArbitraryAxis=[0 0 1]  PositionTargetRotationSequenceAxes=FollowerAxes  PositionTargetRotationSequence=XYX  PositionTargetRotationSequenceAngles=[0 0 0]  PositionTargetRotationSequenceAnglesUnits=deg  PositionTargetRotationMatrix=[1 0 0;0 1 0;0 0 1]  PositionTargetQuaternion=[1 0 0 0]  VelocityTargetSpecify=off  VelocityTargetPriority=High  VelocityTargetValue=[0 0 0]  VelocityTargetValueUnits=deg/s  VelocityTargetInFollowerFrame=on  EqPosRotationMethod=None  EqPosFollAlignAxisA=+X  EqPosBaseAlignAxisA=+Y  EqPosFollAlignAxisB=+Y  EqPosBaseAlignAxisB=+Z  EqPosRotationStandardAxis=+Z  EqPosRotationAngle=0  EqPosRotationAngleUnits=deg  EqPosRotationArbitraryAxis=[0 0 1]  EqPosRotationSequenceAxes=FollowerAxes  EqPosRotationSequence=XYX  EqPosRotationSequenceAngles=[0 0 0]  EqPosRotationSequenceAnglesUnits=deg  EqPosRotationMatrix=[1 0 0;0 1 0;0 0 1]  EqPosQuaternion=[1 0 0 0]  SpringStiffness=Params.Stiffness  SpringStiffnessUnits=N*m/deg  DampingCoefficient=Params.Damping  DampingCoefficientUnits=N*m/(deg/s)  LowerLimitSpecify=off  LowerLimitBound=15  LowerLimitBoundUnits=deg  LowerLimitStiffness=1e4  LowerLimitStiffnessUnits=N*m/deg  LowerLimitDamping=10  LowerLimitDampingUnits=N*m/(deg/s)  LowerLimitTransitionRegionWidth=0.1  LowerLimitTransitionRegionWidthUnits=deg  UpperLimitSpecify=off  UpperLimitBound=45  UpperLimitBoundUnits=deg  UpperLimitStiffness=1e4  UpperLimitStiffnessUnits=N*m/deg  UpperLimitDamping=10  UpperLimitDampingUnits=N*m/(deg/s)  UpperLimitTransitionRegionWidth=0.1  UpperLimitTransitionRegionWidthUnits=deg  TorqueActuationMode=NoTorque  ActuateTorqueX=off  ActuateTorqueY=off  ActuateTorqueZ=off  ActuateTorque=off  ActuationFrame=BaseFrame  SensePosition=on  SenseVelocityX=off  SenseVelocityY=off  SenseVelocityZ=off  SenseVelocity=off  SenseAccelerationX=off  SenseAccelerationY=off  SenseAccelerationZ=off  SenseAcceleration=off  SenseLowerLimitTorqueMag=off  SenseUpperLimitTorqueMag=off  SensingFrame=BaseFrame
  Fixed one : PMIOPort  Side=Left
  base : PMIOPort  Port=2  Side=Right
  q : Outport
  wires:
  PS-Simulink Converter/1 -> Quaternions to Rotation Angles/1
  PS-Simulink Converter1/1 -> Quaternions to Rotation Angles1/1
  PS-Simulink Converter2/1 -> Quaternions to Rotation Angles2/1
  PS-Simulink Converter3/1 -> Quaternions to Rotation Angles3/1
  PS-Simulink Converter5/1 -> Quaternions to Rotation Angles5/1
  PS-Simulink Converter4/1 -> Quaternions to Rotation Angles4/1
  Mux/1 -> q/1
  Plate_2/1(Pos_Plate2) -> Plate_6/7(Pos_Plate2), Plate_5/7(Pos_Plate2), Plate_4/7(Pos_Plate2), Plate_3/7(Pos_Plate2), Plate_1/9(Pos_Plate2)
  Plate_2/2(M2) -> Plate_6/8(M2), Plate_5/8(M2), Plate_4/8(M2), Plate_3/8(M2), Plate_1/10(M2)
  Plate_1/2(M1) -> Plate_6/10(M1), Plate_5/10(M1), Plate_4/10(M1), Plate_3/10(M1), Plate_2/10(M1)
  Plate_1/1(Pos_Plate1) -> Plate_6/9(Pos_Plate1), Plate_5/9(Pos_Plate1), Plate_4/9(Pos_Plate1), Plate_3/9(Pos_Plate1), Plate_2/9(Pos_Plate1)
  Plate_3/2(M3) -> Plate_6/6(M3), Plate_5/6(M3), Plate_4/6(M3), Plate_2/8(M3), Plate_1/8(M3)
  Plate_3/1(Pos_Plate3) -> Plate_6/5(Pos_Plate3), Plate_5/5(Pos_Plate3), Plate_4/5(Pos_Plate3), Plate_2/7(Pos_Plate3), Plate_1/7(Pos_Plate3)
  Plate_4/2(M4) -> Plate_6/4(M4), Plate_5/4(M4), Plate_3/6(M4), Plate_2/6(M4), Plate_1/6(M4)
  Plate_4/1(Pos_Plate4) -> Plate_6/3(Pos_Plate4), Plate_5/3(Pos_Plate4), Plate_3/5(Pos_Plate4), Plate_2/5(Pos_Plate4), Plate_1/5(Pos_Plate4)
  Plate_5/2(M5) -> Plate_6/2(M5), Plate_4/4(M5), Plate_3/4(M5), Plate_2/4(M5), Plate_1/4(M5)
  Plate_5/1(Pos_Plate5) -> Plate_6/1(Pos_Plate5), Plate_4/3(Pos_Plate5), Plate_3/3(Pos_Plate5), Plate_2/3(Pos_Plate5), Plate_1/3(Pos_Plate5)
  Plate_6/2(M6) -> Plate_5/2(M6), Plate_4/2(M6), Plate_3/2(M6), Plate_2/2(M6), Plate_1/2(M6)
  Plate_6/1(Pos_Plate6) -> Plate_5/1(Pos_Plate6), Plate_4/1(Pos_Plate6), Plate_3/1(Pos_Plate6), Plate_2/1(Pos_Plate6), Plate_1/1(Pos_Plate6)
  Quaternions to Rotation Angles/1 -> Mux/1
  Quaternions to Rotation Angles1/1 -> Mux/2
  Quaternions to Rotation Angles2/1 -> Mux/3
  Quaternions to Rotation Angles3/1 -> Mux/4
  Quaternions to Rotation Angles4/1 -> Mux/5
  Quaternions to Rotation Angles5/1 -> Mux/6
  Source_Moment/1 -> Plate_6/12(Source_Moment), Plate_5/12(Source_Moment), Plate_4/12(Source_Moment), Plate_3/12(Source_Moment), Plate_2/12(Source_Moment), Plate_1/12(Source_Moment)
  Source_Pos/1 -> Plate_6/11(Source_Pos), Plate_5/11(Source_Pos), Plate_4/11(Source_Pos), Plate_3/11(Source_Pos), Plate_2/11(Source_Pos), Plate_1/11(Source_Pos)
  connections:
  Rigid Transform11/RConn1 -- Plate_6/RConn1
  Spherical Joint1/LConn1 -- Rigid Transform3/RConn1
  Spherical Joint5/LConn1 -- Rigid Transform12/RConn1
  Rigid Transform2/LConn1 -- Spherical Joint/RConn1
  Rigid Transform11/LConn1 -- Spherical Joint5/RConn1
  Rigid Transform10/RConn1 -- Plate_5/RConn1
  Rigid Transform10/LConn1 -- Spherical Joint4/RConn1
  Rigid Transform4/LConn1 -- Spherical Joint1/RConn1
  Rigid Transform8/RConn1 -- Plate_4/RConn1
  Spherical Joint4/LConn1 -- Rigid Transform9/RConn1
  Plate_4/LConn1 -- Rigid Transform9/LConn1
  Spherical Joint3/LConn1 -- Rigid Transform7/RConn1
  Rigid Transform6/RConn1 -- Plate_3/RConn1
  Rigid Transform8/LConn1 -- Spherical Joint3/RConn1
  Plate_3/LConn1 -- Rigid Transform7/LConn1
  Plate_0/LConn1 -- Rigid Transform1/LConn1
  Spherical Joint/LConn1 -- Rigid Transform1/RConn1
  Plate_2/LConn1 -- Rigid Transform5/LConn1
  Plate_1/LConn1 -- Rigid Transform3/LConn1
  Plate_5/LConn1 -- Rigid Transform12/LConn1
  Rigid Transform4/RConn1 -- Plate_2/RConn1
  Spherical Joint2/LConn1 -- Rigid Transform5/RConn1
  Rigid Transform6/LConn1 -- Spherical Joint2/RConn1
  Rigid Transform2/RConn1 -- Plate_1/RConn1
  Plate_6/LConn1 -- Fixed one/RConn1
  Spherical Joint/RConn2 -- PS-Simulink Converter/LConn1
  Spherical Joint1/RConn2 -- PS-Simulink Converter1/LConn1
  Spherical Joint2/RConn2 -- PS-Simulink Converter2/LConn1
  Spherical Joint3/RConn2 -- PS-Simulink Converter3/LConn1
  Spherical Joint4/RConn2 -- PS-Simulink Converter4/LConn1
  Spherical Joint5/RConn2 -- PS-Simulink Converter5/LConn1
  Rigid Transform13/RConn1 -- Rigid Transform14/LConn1
  base/RConn1 -- Rigid Transform13/LConn1
  Rigid Transform14/RConn1 -- Plate_0/RConn1

== system Copy_of_tests/Multi-Arm system/Single_Arm 1/Plate_0 ==
  Brick Solid : sm_lib/Body Elements/Brick Solid  BrickDimensions=[Params.LinkWidth Params.LinkThickness Params.LinkLength]  BrickDimensionsUnits=m  ExportEntireGeometry=off  InertiaType=CalculateFromGeometry  BasedOnType=Density  Density=1000  DensityUnits=kg/m^3  Mass=1  MassUnits=kg  CenterOfMass=[0 0 0]  CenterOfMassUnits=m  MomentsOfInertia=[1 1 1]  MomentsOfInertiaUnits=kg*m^2  ProductsOfInertia=[0 0 0]  ProductsOfInertiaUnits=kg*m^2  GraphicType=FromGeometry  MarkerShape=Sphere  MarkerSize=10  GraphicVisPropType=SimpleVisualProperties  GraphicDiffuseColor=[0.5 0.5 0.5]  GraphicOpacity=0.5  GraphicSpecularColor=[0.5 0.5 0.5 1.0]  GraphicAmbientColor=[0.15 0.15 0.15 1.0]  GraphicEmissiveColor=[0.0 0.0 0.0 1.0]  GraphicShininess=75  DoExposeReferenceFrame=on  SerializedFrames=<Frames><Frame><Id>Frame1</Id><Value><Name>F1</Name><Origin><Source>GeometricFeature</Source><FeatureName>-x -y curve</FeatureName></Origin><PrimaryAxis><DefinedDirection>+Z</DefinedDirection><Source>ReferenceFrame</Source><SourceDirection>+Z</SourceDirection><FeatureName></FeatureName></PrimaryAxis><SecondaryAxis><DefinedDirection>+X</DefinedDirection><Source>ReferenceFrame</Source><SourceDirection>+X</SourceDirection><FeatureName></FeatureName></SecondaryAxis></Value></Frame><Frame><Id>Frame2</Id><Value><Name>F2</Name><Origin><Source>GeometricFeature</Source><FeatureName>+x -y curve</FeatureName></Origin><PrimaryAxis><DefinedDirection>+Z</DefinedDirection><Source>ReferenceFrame</Source><SourceDirection>+Z</SourceDirection><FeatureName></FeatureName></PrimaryAxis><SecondaryAxis><DefinedDirection>+X</DefinedDirection><Source>ReferenceFrame</Source><SourceDirection>+X</SourceDirection><FeatureName></FeatureName></SecondaryAxis></Value></Frame></Frames>
  Fixed one : PMIOPort  Side=Left
  base : PMIOPort  Port=2  Side=Right
  connections:
  base/RConn1 -- Brick Solid/LConn1
  Brick Solid/LConn2 -- Fixed one/RConn1
